simulink model "Lab1_parameter_estimation_student"  (R2024b)
settings: Solver=FixedStepAuto  StartTime=0.0  StopTime=10  FixedStep=0.001  RelTol=1e-3
values from neighbouring files (symbols this model uses):
  motor_B = 0.00010542    [Estimation_para.m]    (also in constant_motor.m = 0.00019808)
  motor_Eff = 0.95021    [Estimation_para.m]    (also in constant_motor.m = 0.93165)
  motor_J = 1.6624e-05    [Estimation_para.m]    (also in constant_motor.m = 2.8952e-05)
  motor_Ke = 0.042353    [Estimation_para.m]    (also in constant_motor.m = 0.044514)
undefined symbols (not defined in the file or in its folder): motor_L, motor_R
libraries: simulink x7
settings Model: Creator=tanawatp  LastModifiedBy=FREED
settings RTWCC: GPUComputeCapability=3.5

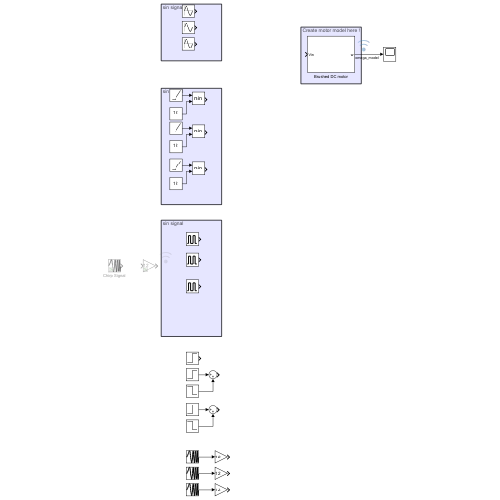
[thumbnail: Simulink's stored preview of the top-level diagram]
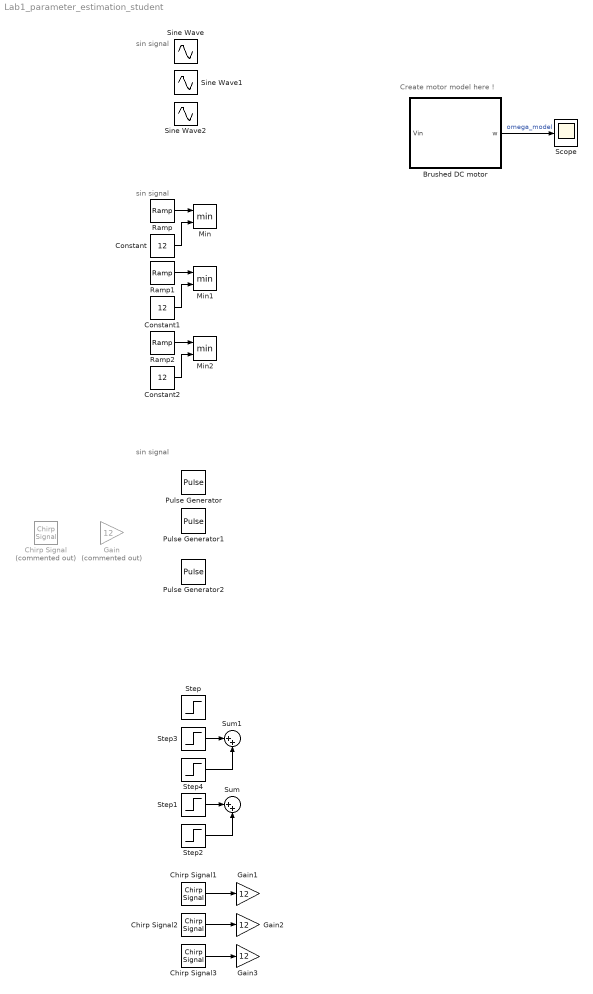
== system Lab1_parameter_estimation_student ==
  note: sin signal
  note: Create motor model here !
  note: sin signal
  note: sin signal
  Brushed DC motor : Subsystem
  Chirp Signal : simulink/Sources/Chirp Signal  Commented=on  f1=0.1  T=40  f2=5
  Chirp Signal1 : simulink/Sources/Chirp Signal  f1=0.1  T=10  f2=1
  Chirp Signal2 : simulink/Sources/Chirp Signal  f1=1  T=10  f2=5
  Chirp Signal3 : simulink/Sources/Chirp Signal  f1=0.1  T=10  f2=0.5
  Constant : Constant  Value=12
  Constant1 : Constant  Value=12
  Constant2 : Constant  Value=12
  Gain : Gain  Commented=on  Gain=12
  Gain1 : Gain  Gain=12
  Gain2 : Gain  Gain=12
  Gain3 : Gain  Gain=12
  Min : MinMax  Inputs=2
  Min1 : MinMax  Inputs=2
  Min2 : MinMax  Inputs=2
  Pulse Generator : DiscretePulseGenerator  PulseType=Time based  Amplitude=12  Period=10  PulseWidth=50
  Pulse Generator1 : DiscretePulseGenerator  PulseType=Time based  Amplitude=12  Period=5  PulseWidth=50
  Pulse Generator2 : DiscretePulseGenerator  PulseType=Time based  Amplitude=12  Period=2.5  PulseWidth=50
  Ramp : simulink/Sources/Ramp  slope=1.2  start=0  InitialOutput=0
  Ramp1 : simulink/Sources/Ramp  slope=2.4  start=0  InitialOutput=0
  Ramp2 : simulink/Sources/Ramp  slope=3.6  start=0  InitialOutput=0
  Scope : Scope
  Sine Wave : Sin  Amplitude=12  Frequency=2*pi*0.1  SampleTime=0
  Sine Wave1 : Sin  Amplitude=12  Frequency=2*pi*1  SampleTime=0
  Sine Wave2 : Sin  Amplitude=12  Frequency=2*pi*2  SampleTime=0
  Step : Step  Time=5  Before=6  After=12  SampleTime=0
  Step1 : Step  Time=5  Before=6  After=12  SampleTime=0
  Step2 : Step  Time=8  After=-24  SampleTime=0
  Step3 : Step  Time=5  Before=6  After=12  SampleTime=0
  Step4 : Step  Time=8  After=-6  SampleTime=0
  Sum : Sum  Inputs=|++
  Sum1 : Sum  Inputs=|++
  wires:
  Brushed DC motor/1(w) -> Scope/1  "omega_model"
  Ramp/1 -> Min/1
  Constant/1 -> Min/2
  Ramp1/1 -> Min1/1
  Constant1/1 -> Min1/2
  Constant2/1 -> Min2/2
  Ramp2/1 -> Min2/1
  Step1/1 -> Sum/1
  Step4/1 -> Sum1/2
  Step3/1 -> Sum1/1
  Step2/1 -> Sum/2
  Chirp Signal1/1 -> Gain1/1
  Chirp Signal2/1 -> Gain2/1
  Chirp Signal3/1 -> Gain3/1

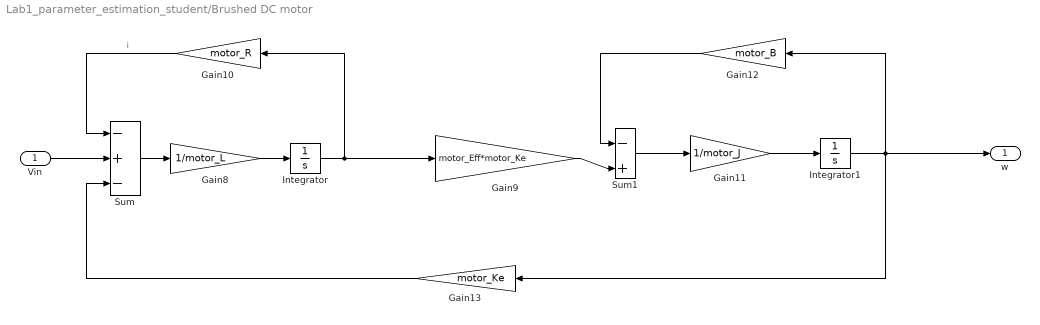
== system Lab1_parameter_estimation_student/Brushed DC motor ==
  Vin : Inport
  Gain10 : Gain  Gain=motor_R
  Gain11 : Gain  Gain=1/motor_J
  Gain12 : Gain  Gain=motor_B
  Gain13 : Gain  Gain=motor_Ke
  Gain8 : Gain  Gain=1/motor_L
  Gain9 : Gain  Gain=motor_Eff*motor_Ke
  Integrator : Integrator
  Integrator1 : Integrator
  Sum : Sum  Inputs=-+-
  Sum1 : Sum  Inputs=-|+|
  w : Outport
  wires:
  Vin/1 -> Sum/2
  Sum/1 -> Gain8/1
  Gain8/1 -> Integrator/1
  Integrator/1 -> Gain9/1, Gain10/1
  Gain10/1 -> Sum/1  "i"
  Sum1/1 -> Gain11/1
  Integrator1/1 -> Gain13/1, Gain12/1, w/1
  Gain12/1 -> Sum1/1
  Gain11/1 -> Integrator1/1
  Gain9/1 -> Sum1/2
  Gain13/1 -> Sum/3
